simulink model "wave"  (R2016b)
settings: Solver=VariableStepAuto  StartTime=0.0  StopTime=10.0  RelTol=1e-3
libraries: simulink x1
settings Model: Creator=charAn  LastModifiedBy=charAn

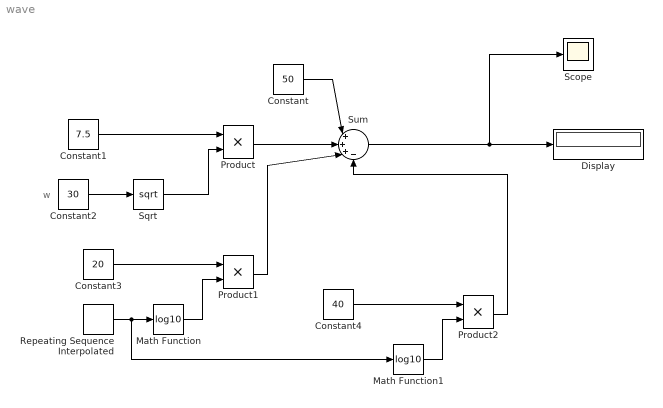
== system wave ==
  note: w
  Constant : Constant  Value=50
  Constant1 : Constant  Value=7.5
  Constant2 : Constant  Value=30
  Constant3 : Constant  Value=20
  Constant4 : Constant  Value=40
  Display : Display
  Math Function : Math  Operator=log10  SaturateOnIntegerOverflow=on
  Math Function1 : Math  Operator=log10  SaturateOnIntegerOverflow=on
  Product : Product
  Product1 : Product
  Product2 : Product
  Repeating Sequence Interpolated : simulink/Sources/Repeating Sequence Interpolated  OutValues=[0 200 10200 20200 30200 40200 50200 60200 70200 80200 90200 100200 110200 120200 130200 140200 150200 160200 170200 180200 190200 200200]  TimeValues=[0 200 10200 20200 30200 40200 50200 60200 70200 80200 90200 100200 110200 120200 130200 140200 150200 160200 170200 180200 190200 200200]  LookUpMeth=Interpolation-Use End Values  tsamp=0.01  OutMin=[]  OutMax=[]  OutDataTypeStr=double  OutputDataTypeScalingMode=double  OutDataType=fixdt(0,8)  OutScaling=2^-10
  Scope : Scope
  Sqrt : Sqrt  SaturateOnIntegerOverflow=on
  Sum : Sum  Inputs=|+++-
  wires:
  Constant2/1 -> Sqrt/1
  Constant1/1 -> Product/1
  Sqrt/1 -> Product/2
  Product/1 -> Sum/2
  Constant/1 -> Sum/1
  Constant3/1 -> Product1/1
  Math Function/1 -> Product1/2
  Product1/1 -> Sum/3
  Repeating Sequence Interpolated/1 -> Math Function1/1, Math Function/1
  Constant4/1 -> Product2/1
  Math Function1/1 -> Product2/2
  Product2/1 -> Sum/4
  Sum/1 -> Scope/1, Display/1
